simulink model "PMSM"  (R2014b)
settings: Solver=ode1  StartTime=0.0  StopTime=4  FixedStep=0.00001  RelTol=1e-3
values from neighbouring files (symbols this model uses):
  f = 50    [parameter.mat]
  J = 0.089    [parameter.mat]
  Ld = 0.0085    [parameter.mat]
  Lq = 0.0085    [parameter.mat]
  n_soll = 3000    [parameter.mat]
  p = 4    [parameter.mat]
  Psi_pm = 0.175    [parameter.mat]
  R1 = 0.2    [parameter.mat]
settings Model: Creator=benjamin  LastModifiedBy=benjamin

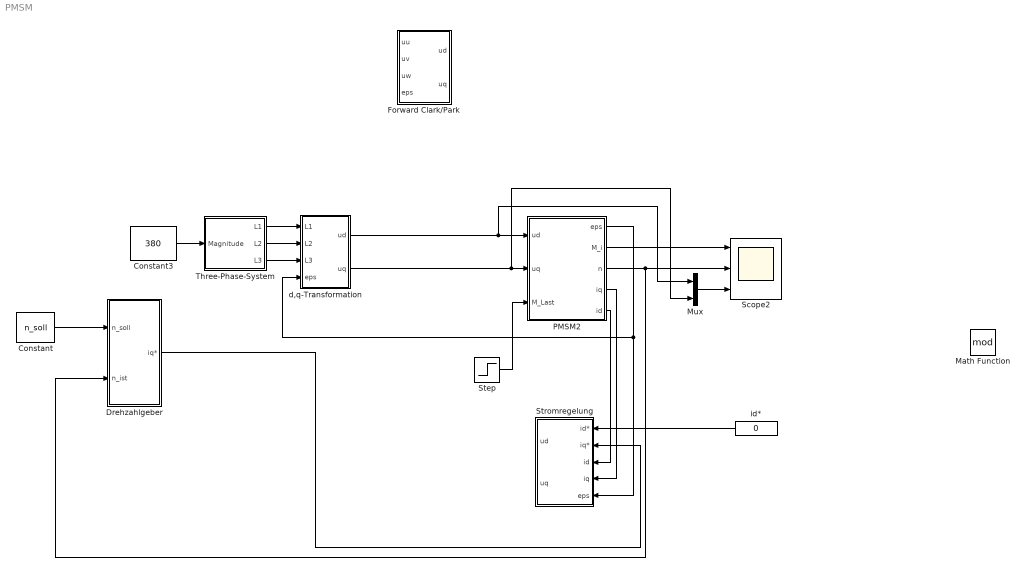
== system PMSM ==
  Constant : Constant  Value=n_soll
  Constant3 : Constant  Value=380
  Drehzahlgeber : Subsystem
  Forward Clark/Park : Subsystem
  Math Function : Math  Operator=mod  SaturateOnIntegerOverflow=on
  Mux : Mux  Inputs=2
  PMSM2 : Subsystem
  Scope2 : Scope  NumInputPorts=3
      settings: TimeRange=1  YMin=-2~-10000~-40000  YMax=18~15000~60000  SaveName=ScopeData2
  Step : Step  After=10  SampleTime=0
  Stromregelung : Subsystem
  Three-Phase-System : Subsystem
  d,q-Transformation : Subsystem
  id* : Constant  Value=0
  wires:
  Constant3/1 -> Three-Phase-System/1(Magnitude)
  Mux/1 -> Scope2/3
  Step/1 -> PMSM2/3(M_Last)
  d,q-Transformation/1(ud) -> PMSM2/1(ud), Mux/1
  Three-Phase-System/1(L1) -> d,q-Transformation/1(L1)
  Three-Phase-System/2(L2) -> d,q-Transformation/2(L2)
  Three-Phase-System/3(L3) -> d,q-Transformation/3(L3)
  PMSM2/1(eps) -> Stromregelung/5(eps), d,q-Transformation/4(eps)
  PMSM2/2(M_i) -> Scope2/1
  PMSM2/3(n) -> Scope2/2, Drehzahlgeber/2(n_ist)
  d,q-Transformation/2(uq) -> Mux/2, PMSM2/2(uq)
  PMSM2/4(iq) -> Stromregelung/4(iq)
  PMSM2/5(id) -> Stromregelung/3(id)
  id*/1 -> Stromregelung/1(id*)
  Drehzahlgeber/1(iq*) -> Stromregelung/2(iq*)
  Constant/1 -> Drehzahlgeber/1(n_soll)

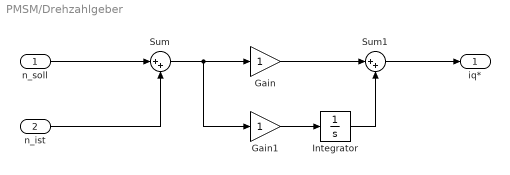
== system PMSM/Drehzahlgeber ==
  n_soll : Inport
  n_ist : Inport  Port=2
  Gain : Gain
  Gain1 : Gain
  Integrator : Integrator
  Sum : Sum  Inputs=|++
  Sum1 : Sum  Inputs=|++
  iq* : Outport
  wires:
  n_soll/1 -> Sum/1
  n_ist/1 -> Sum/2
  Sum/1 -> Gain1/1, Gain/1
  Gain/1 -> Sum1/1
  Gain1/1 -> Integrator/1
  Integrator/1 -> Sum1/2
  Sum1/1 -> iq*/1

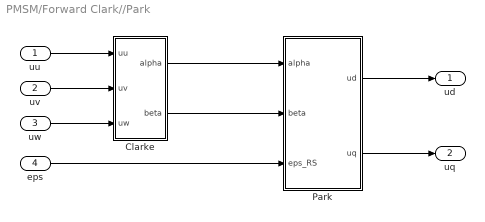
== system PMSM/Forward Clark//Park ==
  uu : Inport
  uv : Inport  Port=2
  uw : Inport  Port=3
  eps : Inport  Port=4
  Clarke : Subsystem
  Park : Subsystem
  ud : Outport
  uq : Outport  Port=2
  wires:
  uw/1 -> Clarke/3(uw)
  uu/1 -> Clarke/1(uu)
  eps/1 -> Park/3(eps_RS)
  Park/1(ud) -> ud/1
  uv/1 -> Clarke/2(uv)
  Park/2(uq) -> uq/1
  Clarke/1(alpha) -> Park/1(alpha)
  Clarke/2(beta) -> Park/2(beta)

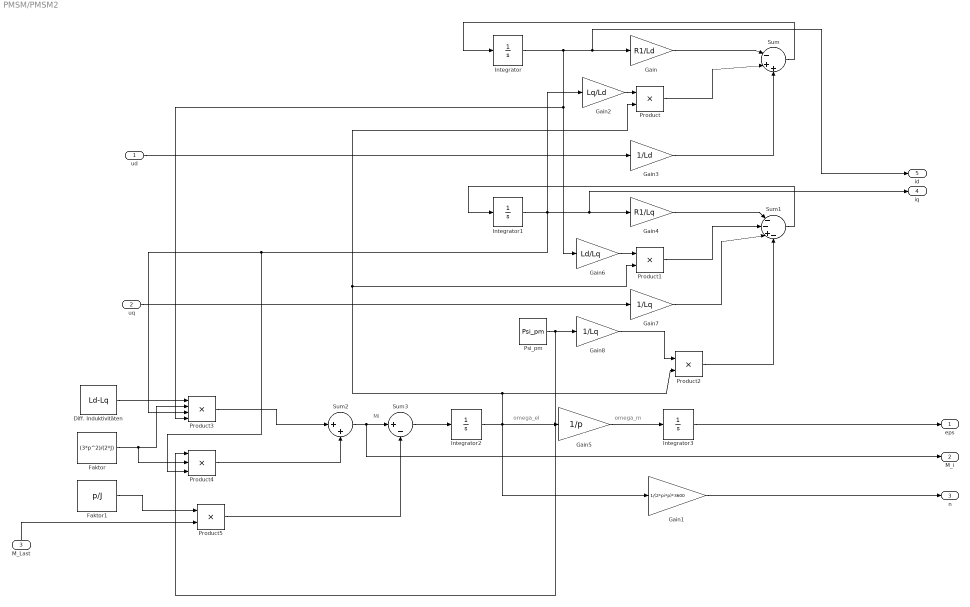
== system PMSM/PMSM2 ==
  note: omega_el
  note: Mi
  note: omega_m
  ud : Inport
  uq : Inport  Port=2
  M_Last : Inport  Port=3
  Diff. Induktivitäten : Constant  Value=Ld-Lq
  Faktor : Constant  Value=(3*p^2)/(2*J)
  Faktor1 : Constant  Value=p/J
  Gain : Gain  Gain=R1/Ld
  Gain1 : Gain  Gain=1/(2*pi*p)*3600
  Gain2 : Gain  Gain=Lq/Ld
  Gain3 : Gain  Gain=1/Ld
  Gain4 : Gain  Gain=R1/Lq
  Gain5 : Gain  Gain=1/p
  Gain6 : Gain  Gain=Ld/Lq
  Gain7 : Gain  Gain=1/Lq
  Gain8 : Gain  Gain=1/Lq
  Integrator{,1..3} (4 alike) : Integrator
  Product{,1..2,5} (4 alike) : Product
  Product3 : Product  Inputs=4
  Product4 : Product  Inputs=3
  Psi_pm : Constant  Value=Psi_pm
  Sum : Sum  Inputs=|-++
  Sum1 : Sum  Inputs=|--+-
  Sum2 : Sum  Inputs=|++
  Sum3 : Sum  Inputs=|+-
  eps : Outport
  M_i : Outport  Port=2
  n : Outport  Port=3
  iq : Outport  Port=4
  id : Outport  Port=5
  wires:
  Sum1/1 -> Integrator1/1
  Gain/1 -> Sum/1
  Product/1 -> Sum/2
  Gain3/1 -> Sum/3
  Gain2/1 -> Product/1
  Integrator/1 -> Gain6/1, Product3/4, id/1, Gain/1
  Integrator1/1 -> Product4/3, Product3/3, Gain2/1, iq/1, Gain4/1
  Product1/1 -> Sum1/2
  Gain7/1 -> Sum1/3
  uq/1 -> Gain7/1
  Faktor/1 -> Product4/2, Product3/2
  Product4/1 -> Sum2/2
  Gain4/1 -> Sum1/1
  Sum/1 -> Integrator/1
  Diff. Induktivitäten/1 -> Product3/1
  Gain8/1 -> Product2/1
  Psi_pm/1 -> Product4/1, Gain8/1
  Product3/1 -> Sum2/1
  Product2/1 -> Sum1/4
  Faktor1/1 -> Product5/1
  M_Last/1 -> Product5/2
  Sum2/1 -> Sum3/1, M_i/1
  ud/1 -> Gain3/1
  Gain6/1 -> Product1/1
  Integrator2/1 -> Gain1/1, Gain5/1, Product2/2, Product/2, Product1/2
  Integrator3/1 -> eps/1
  Sum3/1 -> Integrator2/1
  Product5/1 -> Sum3/2
  Gain1/1 -> n/1
  Gain5/1 -> Integrator3/1

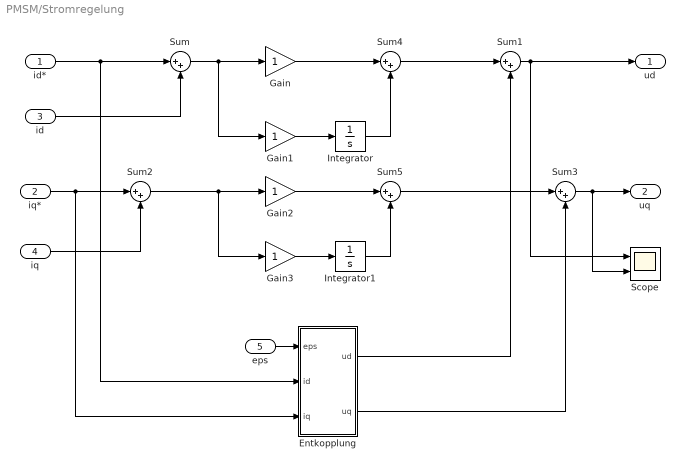
== system PMSM/Stromregelung ==
  id* : Inport
  iq* : Inport  Port=2
  id : Inport  Port=3
  iq : Inport  Port=4
  eps : Inport  Port=5
  Entkopplung : Subsystem
  Gain{,1..3} (4 alike) : Gain
  Integrator : Integrator
  Integrator1 : Integrator
  Scope : Scope  NumInputPorts=2
      settings: TimeRange=5  YMin=-1.3~-5  YMax=0~5
  Sum{,1..5} (6 alike) : Sum  Inputs=|++
  ud : Outport
  uq : Outport  Port=2
  wires:
  Sum3/1 -> Scope/2, uq/1
  Entkopplung/1(ud) -> Sum1/2
  iq*/1 -> Entkopplung/3(iq), Sum2/1
  id*/1 -> Entkopplung/2(id), Sum/1
  eps/1 -> Entkopplung/1(eps)
  id/1 -> Sum/2
  Entkopplung/2(uq) -> Sum3/2
  iq/1 -> Sum2/2
  Sum1/1 -> ud/1, Scope/1
  Sum/1 -> Gain1/1, Gain/1
  Gain/1 -> Sum4/1
  Gain1/1 -> Integrator/1
  Integrator/1 -> Sum4/2
  Sum4/1 -> Sum1/1
  Sum2/1 -> Gain3/1, Gain2/1
  Gain2/1 -> Sum5/1
  Gain3/1 -> Integrator1/1
  Integrator1/1 -> Sum5/2
  Sum5/1 -> Sum3/1

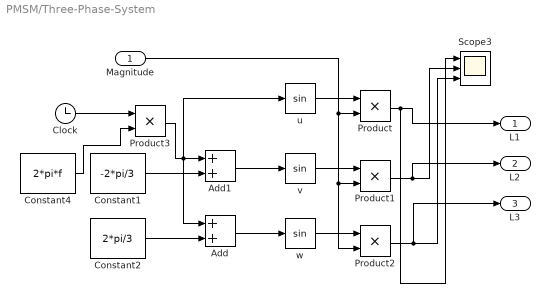
== system PMSM/Three-Phase-System ==
  Magnitude : Inport
  Add : Sum
  Add1 : Sum
  Clock : Clock
  Constant1 : Constant  Value=-2*pi/3
  Constant2 : Constant  Value=2*pi/3
  Constant4 : Constant  Value=2*pi*f
  Product{,1..3} (4 alike) : Product
  Scope3 : Scope  NumInputPorts=3
      settings: YMin=-5~-5~-5  YMax=5~5~5
  u : Trigonometry
  v : Trigonometry
  w : Trigonometry
  L1 : Outport
  L2 : Outport  Port=2
  L3 : Outport  Port=3
  wires:
  Constant2/1 -> Add/2
  Add/1 -> w/1
  Add1/1 -> v/1
  Constant1/1 -> Add1/2
  Product2/1 -> L3/1, Scope3/3
  Product/1 -> L1/1, Scope3/1
  w/1 -> Product2/1
  Product3/1 -> Add/1, Add1/1, u/1
  Clock/1 -> Product3/1
  Product1/1 -> L2/1, Scope3/2
  Constant4/1 -> Product3/2
  Magnitude/1 -> Product2/2, Product1/2, Product/2
  u/1 -> Product/1
  v/1 -> Product1/1

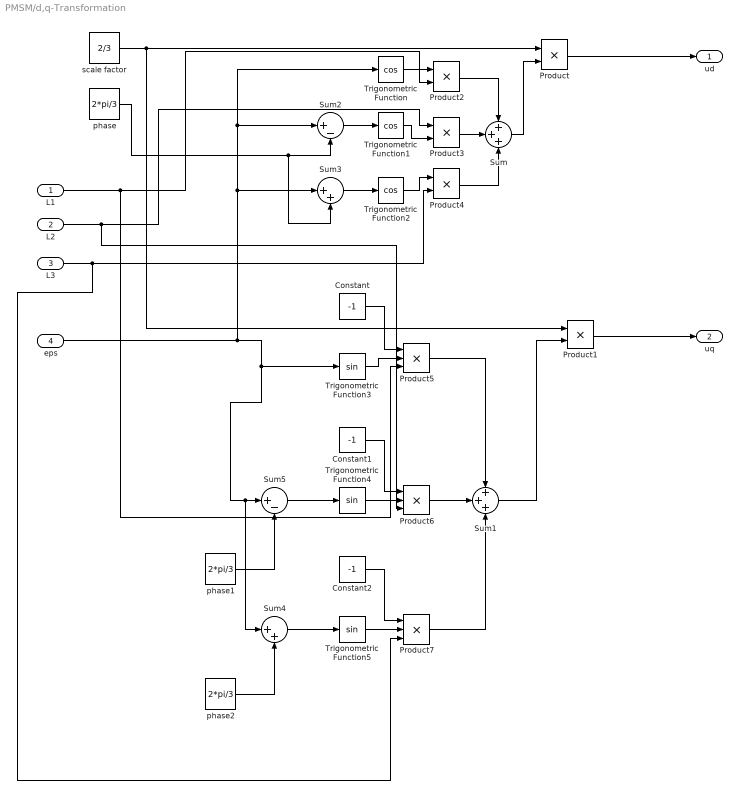
== system PMSM/d,q-Transformation ==
  L1 : Inport
  L2 : Inport  Port=2
  L3 : Inport  Port=3
  eps : Inport  Port=4
  Constant : Constant  Value=-1
  Constant1 : Constant  Value=-1
  Constant2 : Constant  Value=-1
  Product{,1..4} (5 alike) : Product
  Product5 : Product  Inputs=3
  Product6 : Product  Inputs=3
  Product7 : Product  Inputs=3
  Sum : Sum  Inputs=+++
  Sum1 : Sum  Inputs=+++
  Sum2 : Sum  Inputs=|+-
  Sum3 : Sum  Inputs=|++
  Sum4 : Sum  Inputs=|++
  Sum5 : Sum  Inputs=|+-
  Trigonometric Function : Trigonometry  Operator=cos
  Trigonometric Function1 : Trigonometry  Operator=cos
  Trigonometric Function2 : Trigonometry  Operator=cos
  Trigonometric Function3 : Trigonometry
  Trigonometric Function4 : Trigonometry
  Trigonometric Function5 : Trigonometry
  phase : Constant  Value=2*pi/3
  phase1 : Constant  Value=2*pi/3
  phase2 : Constant  Value=2*pi/3
  scale factor : Constant  Value=2/3
  ud : Outport
  uq : Outport  Port=2
  wires:
  Sum1/1 -> Product1/2
  Sum/1 -> Product/2
  scale factor/1 -> Product1/1, Product/1
  Product5/1 -> Sum1/1
  Product7/1 -> Sum1/3
  eps/1 -> Sum4/1, Sum5/1, Trigonometric Function3/1, Sum3/1, Sum2/1, Trigonometric Function/1
  Product/1 -> ud/1
  Sum2/1 -> Trigonometric Function1/1
  phase/1 -> Sum3/2, Sum2/2
  L1/1 -> Product5/3, Product2/2
  Trigonometric Function/1 -> Product2/1
  Product2/1 -> Sum/1
  Product3/1 -> Sum/2
  L2/1 -> Product6/3, Product3/1
  Trigonometric Function1/1 -> Product3/2
  Sum3/1 -> Trigonometric Function2/1
  Trigonometric Function2/1 -> Product4/1
  L3/1 -> Product4/2, Product7/3
  Product4/1 -> Sum/3
  Product1/1 -> uq/1
  Constant/1 -> Product5/1
  Trigonometric Function3/1 -> Product5/2
  Constant1/1 -> Product6/1
  Trigonometric Function4/1 -> Product6/2
  Constant2/1 -> Product7/1
  Trigonometric Function5/1 -> Product7/2
  Product6/1 -> Sum1/2
  phase1/1 -> Sum5/2
  phase2/1 -> Sum4/2
  Sum5/1 -> Trigonometric Function4/1
  Sum4/1 -> Trigonometric Function5/1

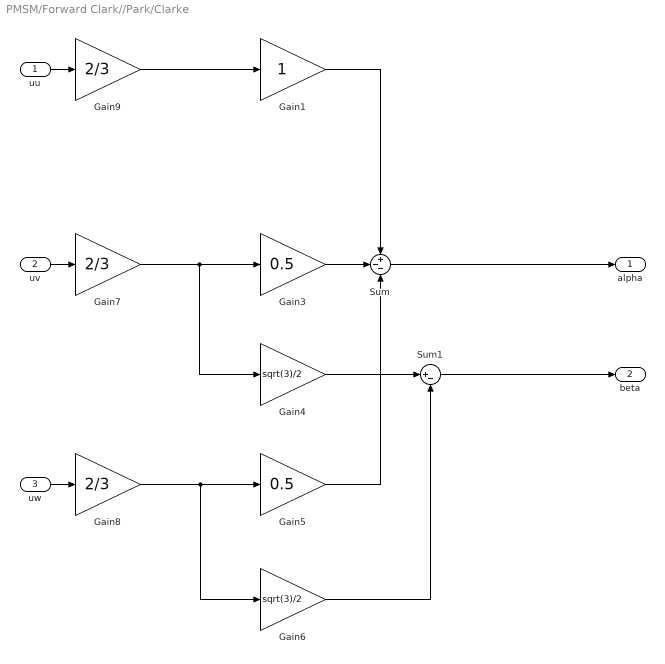
== system PMSM/Forward Clark//Park/Clarke ==
  uu : Inport
  uv : Inport  Port=2
  uw : Inport  Port=3
  Gain1 : Gain
  Gain3 : Gain  Gain=0.5
  Gain4 : Gain  Gain=sqrt(3)/2
  Gain5 : Gain  Gain=0.5
  Gain6 : Gain  Gain=sqrt(3)/2
  Gain7 : Gain  Gain=2/3
  Gain8 : Gain  Gain=2/3
  Gain9 : Gain  Gain=2/3
  Sum : Sum  Inputs=+--
  Sum1 : Sum  Inputs=|+-
  alpha : Outport
  beta : Outport  Port=2
  wires:
  Gain1/1 -> Sum/1
  Gain5/1 -> Sum/3
  uw/1 -> Gain8/1
  Gain3/1 -> Sum/2
  Gain7/1 -> Gain4/1, Gain3/1
  Gain9/1 -> Gain1/1
  Gain8/1 -> Gain6/1, Gain5/1
  Sum/1 -> alpha/1
  Sum1/1 -> beta/1
  uv/1 -> Gain7/1
  uu/1 -> Gain9/1
  Gain4/1 -> Sum1/1
  Gain6/1 -> Sum1/2

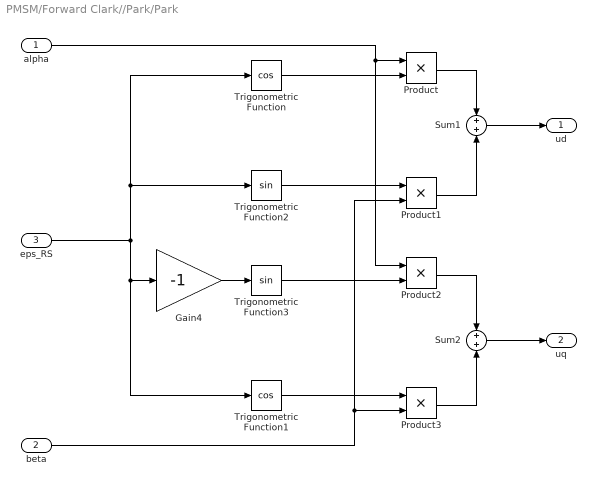
== system PMSM/Forward Clark//Park/Park ==
  alpha : Inport
  beta : Inport  Port=2
  eps_RS : Inport  Port=3
  Gain4 : Gain  Gain=-1
  Product{,1..3} (4 alike) : Product
  Sum1 : Sum
  Sum2 : Sum
  Trigonometric Function : Trigonometry  Operator=cos
  Trigonometric Function1 : Trigonometry  Operator=cos
  Trigonometric Function2 : Trigonometry
  Trigonometric Function3 : Trigonometry
  ud : Outport
  uq : Outport  Port=2
  wires:
  Sum2/1 -> uq/1
  Product2/1 -> Sum2/1
  Product1/1 -> Sum1/2
  eps_RS/1 -> Trigonometric Function2/1, Trigonometric Function/1, Gain4/1, Trigonometric Function1/1
  Trigonometric Function/1 -> Product/2
  alpha/1 -> Product2/1, Product/1
  Sum1/1 -> ud/1
  Trigonometric Function1/1 -> Product3/1
  beta/1 -> Product3/2, Product1/2
  Product/1 -> Sum1/1
  Trigonometric Function2/1 -> Product1/1
  Trigonometric Function3/1 -> Product2/2
  Product3/1 -> Sum2/2
  Gain4/1 -> Trigonometric Function3/1

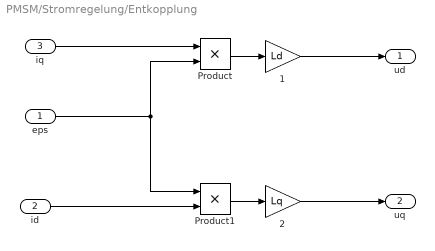
== system PMSM/Stromregelung/Entkopplung ==
  eps : Inport
  id : Inport  Port=2
  iq : Inport  Port=3
  1 : Gain  Gain=Ld
  2 : Gain  Gain=Lq
  Product : Product  RndMeth=Zero
  Product1 : Product  RndMeth=Zero
  ud : Outport
  uq : Outport  Port=2
  wires:
  eps/1 -> Product/2, Product1/1
  Product/1 -> 1/1
  1/1 -> ud/1
  iq/1 -> Product/1
  id/1 -> Product1/2
  Product1/1 -> 2/1
  2/1 -> uq/1
